simulink model "Boeing787_debug"  (R2013a)
settings: Solver=ode23tb  SolverMode=SingleTasking  StartTime=0.0  StopTime=18000  RelTol=1e-3
InitFcn:
  | load('SampleOutput.mat')
  | 
  | load('SampleFuelBurn.mat')
StartFcn:
  | tic
StopFcn:
  | ttt = toc
  | tend = eval(get_param(bdroot,'StopTime'));
  | disp(['Total Simulation Time (s) = ' num2str(ttt) 's']);
  | RTR =  ttt/tend
  | disp(['Simulation Speed is ' num2str(tend/ttt) 'x faster than real-time']);
values from neighbouring files (symbols this model uses):
  FuelBurn = [0 0 0 0 0 0 0 0 0 0 0 0 ... (18249 elements, 1x18249)]    [Benchmark_data1.mat]
undefined symbols (not defined in the file or in its folder): CurrentMission, seed
libraries: PowerFlowLib x20, simulink x14, powerlib_meascontrol x3
(part 17 of 17)

== system Boeing787_debug/Electrical/Generation Unit Sync-Sync4/Generator/Generator Power Loss ==
  Ed : Inport
  Eq : Inport  Port=2
  Id : Inport  Port=3
  Iq : Inport  Port=4
  Te : Inport  Port=5
  w/ws : Inport  Port=6
  Bus Creator : BusCreator  Inputs=6
  Gain1 : Gain  Gain=SB
  Gain2 : Gain  Gain=SB
  Gain3 : Gain  Gain=SB
  Product : Product  RndMeth=Zero
  Product1 : Product  RndMeth=Zero
  Product2 : Product  RndMeth=Zero
  Sum1 : Sum  Inputs=-+
  Sum2 : Sum
  PE : Outport
  PM : Outport  Port=2
  PLOSS : Outport  Port=3
  m : Outport  Port=4
  wires:
  Ed/1 -> [Ed]
  Eq/1 -> [Eq]
  Id/1 -> [Id]
  Iq/1 -> [Iq]
  Te/1 -> [Te]
  w/ws/1 -> [nu]
  [Ed] -> Product/1
  [Id] -> Product/2
  [Eq] -> Product1/1
  [Iq] -> Product1/2
  [Te] -> Product2/1
  [nu] -> Product2/2
  Product/1 -> Sum2/1
  Product1/1 -> Sum2/2
  Sum2/1 -> Sum1/1, Gain1/1
  Product2/1 -> Sum1/2, Gain3/1
  Sum1/1 -> Gain2/1
  [Ed] -> Bus Creator/1  "Vd"
  [Id] -> Bus Creator/2  "Id"
  [Eq] -> Bus Creator/3  "Vq"
  [Iq] -> Bus Creator/4  "Iq"
  [Te] -> Bus Creator/5  "Te"
  [nu] -> Bus Creator/6  "nu"
  Bus Creator/1 -> m/1
  Gain2/1 -> PLOSS/1
  Gain1/1 -> PE/1
  Gain3/1 -> PM/1

== system Boeing787_debug/Electrical/Generation Unit Sync-Sync4/Generator/Stator Voltage ==
  Id : Inport
  Iq : Inport  Port=2
  Eq1 : Inport  Port=3
  Ed1 : Inport  Port=4
  Phi_1d : Inport  Port=5
  Phi_2q : Inport  Port=6
  w/ws : Inport  Port=7
  Temp : Inport  Port=8
  Gain : Gain  Gain=(Xq2 - Xls)/(Xq1 - Xls)
  Gain1 : Gain  Gain=(Xq1 - Xq2)/(Xq1 - Xls)
  Gain2 : Gain  Gain=(Xq2 - Xd2)
  Gain3 : Gain  Gain=(Xd2 - Xls)/(Xd1 - Xls)
  Gain4 : Gain  Gain=(Xd1 - Xd2)/(Xd1 - Xls)
  Gain5 : Gain  Gain=Rs
  Gain6 : Gain  Gain=Xd2
  Gain7 : Gain  Gain=Rs
  Gain8 : Gain  Gain=Xd2
  Product{,1..3,5} (5 alike) : Product  RndMeth=Zero
  Product4 : Product
  Sum : Sum
  Sum1 : Sum  Inputs=+-+
  Sum2 : Sum  Inputs=--+
  Sum3 : Sum  Inputs=-++
  Ed : Outport
  Eq : Outport  Port=2
  wires:
  Iq/1 -> Gain6/1, Product5/2, Gain2/1
  Product5/1 -> Gain7/1
  Product4/1 -> Sum3/1
  Gain5/1 -> Product4/1
  Temp/1 -> Product4/2, Product5/1
  Gain2/1 -> Sum1/3
  Ed1/1 -> Gain/1
  Phi_2q/1 -> Gain1/1
  Eq1/1 -> Gain3/1
  Phi_1d/1 -> Gain4/1
  Gain4/1 -> Sum/2
  Gain3/1 -> Sum/1
  Gain/1 -> Sum1/1
  Gain1/1 -> Sum1/2
  Sum/1 -> Product/1
  Sum1/1 -> Product1/1
  w/ws/1 -> Product1/2, Product/2, Product3/2, Product2/1
  Product/1 -> Sum2/3
  Id/1 -> Gain5/1, Gain8/1
  Gain6/1 -> Product2/2
  Gain8/1 -> Product3/1
  Product1/1 -> Sum3/2
  Product2/1 -> Sum3/3
  Sum3/1 -> Ed/1  "Vd"
  Sum2/1 -> Eq/1  "Vq"
  Product3/1 -> Sum2/1
  Gain7/1 -> Sum2/2

== system Boeing787_debug/Electrical/Generation Unit Sync-Sync5/Exciter/Dynamics ==
  Id : Inport
  Iq : Inport  Port=2
  Efd : Inport  Port=3
  Temp : Inport  Port=4
  Gain : Gain  Gain=Xd1_exc - Xls_exc
  Gain1 : Gain  Gain=(Xd1_exc - Xd2_exc)/(Xd1_exc-Xls_exc)^2
  Gain10 : Gain  Gain=Xq1_exc - Xls_exc
  Gain11 : Gain  Gain=1/Tqo2_exc
  Gain2 : Gain  Gain=Xd_exc - Xd1_exc
  Gain3 : Gain  Gain=1/Tdo1_exc
  Gain4 : Gain  Gain=Xq1_exc - Xls_exc
  Gain5 : Gain  Gain=(Xq1_exc - Xq2_exc)/(Xq1_exc - Xls_exc)^2
  Gain6 : Gain  Gain=Xq_exc - Xq1_exc
  Gain7 : Gain  Gain=1/Tqo1_exc
  Gain8 : Gain  Gain=Xd1_exc - Xls_exc
  Gain9 : Gain  Gain=1/Tdo2_exc
  Integrator{,1..3} (4 alike) : Integrator
  Product{,1..3} (4 alike) : Product
  Sum : Sum  Inputs=++-
  Sum1 : Sum  Inputs=+-
  Sum2 : Sum  Inputs=--+
  Sum3 : Sum  Inputs=+++
  Sum4 : Sum  Inputs=+-
  Sum5 : Sum  Inputs=-+
  Sum6 : Sum  Inputs=--+
  Sum7 : Sum  Inputs=---
  Eq1 : Outport
  Ed1 : Outport  Port=2
  Phi_1d : Outport  Port=3
  Phi_2q : Outport  Port=4
  wires:
  Integrator/1 -> Eq1/1, [Eq1]
  [Id] -> Gain/1
  Gain/1 -> Sum/1
  [Phi_1d] -> Sum/2
  [Eq1] -> Sum/3
  Sum/1 -> Gain1/1
  [Id] -> Sum1/1
  Gain1/1 -> Sum1/2
  Sum1/1 -> Gain2/1
  [Eq1] -> Sum2/1
  Gain2/1 -> Sum2/2
  [Efd] -> Sum2/3
  Sum2/1 -> Gain3/1
  Integrator1/1 -> Ed1/1, [Ed1]
  [Iq] -> Gain4/1
  Gain4/1 -> Sum3/1
  [Phi_2q] -> Sum3/2
  [Ed1] -> Sum3/3
  Sum3/1 -> Gain5/1
  [Iq] -> Sum4/1
  Gain5/1 -> Sum4/2
  Sum4/1 -> Gain6/1
  [Ed1] -> Sum5/1
  Gain6/1 -> Sum5/2
  Sum5/1 -> Gain7/1
  [Id] -> Gain8/1
  Gain8/1 -> Sum6/1
  [Phi_1d] -> Sum6/2
  [Eq1] -> Sum6/3
  Sum6/1 -> Gain9/1
  Integrator2/1 -> [Phi_1d], Phi_1d/1
  [Iq] -> Gain10/1
  Gain10/1 -> Sum7/1
  [Phi_2q] -> Sum7/2
  [Ed1] -> Sum7/3
  Sum7/1 -> Gain11/1
  Integrator3/1 -> [Phi_2q], Phi_2q/1
  Id/1 -> [Id]
  Iq/1 -> [Iq]
  Efd/1 -> [Efd]
  Temp/1 -> [R_temp_delta]
  Gain3/1 -> Product/2
  Product/1 -> Integrator/1
  [R_temp_delta] -> Product/1
  [R_temp_delta] -> Product1/1
  Gain7/1 -> Product1/2
  Product1/1 -> Integrator1/1
  [R_temp_delta] -> Product2/1
  Gain11/1 -> Product2/2
  Product2/1 -> Integrator3/1
  [R_temp_delta] -> Product3/1
  Gain9/1 -> Product3/2
  Product3/1 -> Integrator2/1

== system Boeing787_debug/Electrical/Generation Unit Sync-Sync5/Exciter/Electromagnetic Torque Output Power ==
  note: Torque from Field Winding
  note: Torque from Damper Windings
  Id : Inport
  Iq : Inport  Port=2
  Eq1 : Inport  Port=3
  Ed1 : Inport  Port=4
  Phi_1d : Inport  Port=5
  Phi_2q : Inport  Port=6
  Gain : Gain  Gain=(Xd2_exc - Xls_exc)/(Xd1_exc - Xls_exc)
  Gain1 : Gain  Gain=(Xq2_exc - Xls_exc)/(Xq1_exc - Xls_exc)
  Gain2 : Gain  Gain=(Xd1_exc - Xd2_exc)/(Xd1_exc-Xls_exc)
  Gain3 : Gain  Gain=(Xq1_exc - Xq2_exc)/(Xq1_exc-Xls_exc)
  Gain4 : Gain  Gain=(Xq2_exc - Xd2_exc)
  Product{,1..4} (5 alike) : Product  RndMeth=Zero
  Sum : Sum
  Sum1 : Sum  Inputs=+-+
  Sum2 : Sum
  TE : Outport
  wires:
  Id/1 -> [Id]
  Eq1/1 -> [Eq1]
  Ed1/1 -> [Ed1]
  Phi_1d/1 -> [Phi_1d]
  Phi_2q/1 -> [Phi_2q]
  Iq/1 -> [Iq]
  [Eq1] -> Product/1
  [Iq] -> Product/2
  Product/1 -> Gain/1
  [Ed1] -> Product1/1
  [Id] -> Product1/2
  Product1/1 -> Gain1/1
  [Iq] -> Product2/1
  [Phi_1d] -> Product2/2
  Product2/1 -> Gain2/1
  [Id] -> Product3/1
  [Phi_2q] -> Product3/2
  Product3/1 -> Gain3/1
  [Id] -> Product4/1
  [Iq] -> Product4/2
  Product4/1 -> Gain4/1
  Gain3/1 -> Sum1/2
  Gain2/1 -> Sum1/1
  Gain4/1 -> Sum1/3
  Gain/1 -> Sum/1
  Gain1/1 -> Sum/2
  Sum/1 -> Sum2/1
  Sum1/1 -> Sum2/2
  Sum2/1 -> TE/1

== system Boeing787_debug/Electrical/Generation Unit Sync-Sync5/Exciter/Generator Power Loss ==
  Ed : Inport
  Eq : Inport  Port=2
  Id : Inport  Port=3
  Iq : Inport  Port=4
  Te : Inport  Port=5
  w/ws : Inport  Port=6
  Bus Creator : BusCreator  Inputs=6
  Gain1 : Gain  Gain=SB_exc
  Gain2 : Gain  Gain=SB_exc
  Gain3 : Gain  Gain=SB_exc
  Product : Product  RndMeth=Zero
  Product1 : Product  RndMeth=Zero
  Product2 : Product  RndMeth=Zero
  Sum1 : Sum  Inputs=-+
  Sum2 : Sum
  PE : Outport
  PM : Outport  Port=2
  PLOSS : Outport  Port=3
  m : Outport  Port=4
  wires:
  Ed/1 -> [Ed]
  Eq/1 -> [Eq]
  Id/1 -> [Id]
  Iq/1 -> [Iq]
  Te/1 -> [Te]
  w/ws/1 -> [nu]
  [Ed] -> Product/1
  [Id] -> Product/2
  [Eq] -> Product1/1
  [Iq] -> Product1/2
  [Te] -> Product2/1
  [nu] -> Product2/2
  Product/1 -> Sum2/1
  Product1/1 -> Sum2/2
  Sum2/1 -> Sum1/1, Gain1/1
  Product2/1 -> Sum1/2, Gain3/1
  Sum1/1 -> Gain2/1
  [Ed] -> Bus Creator/1  "Vd"
  [Id] -> Bus Creator/2  "Id"
  [Eq] -> Bus Creator/3  "Vq"
  [Iq] -> Bus Creator/4  "Iq"
  [Te] -> Bus Creator/5  "Te"
  [nu] -> Bus Creator/6  "nu"
  Bus Creator/1 -> m/1
  Gain2/1 -> PLOSS/1
  Gain1/1 -> PE/1
  Gain3/1 -> PM/1

== system Boeing787_debug/Electrical/Generation Unit Sync-Sync5/Exciter/Stator Voltage ==
  Id : Inport
  Iq : Inport  Port=2
  Eq1 : Inport  Port=3
  Ed1 : Inport  Port=4
  Phi_1d : Inport  Port=5
  Phi_2q : Inport  Port=6
  w/ws : Inport  Port=7
  Temp : Inport  Port=8
  Gain : Gain  Gain=(Xq2_exc - Xls_exc)/(Xq1_exc - Xls_exc)
  Gain1 : Gain  Gain=(Xq1_exc - Xq2_exc)/(Xq1_exc - Xls_exc)
  Gain2 : Gain  Gain=(Xq2_exc - Xd2_exc)
  Gain3 : Gain  Gain=(Xd2_exc - Xls_exc)/(Xd1_exc - Xls_exc)
  Gain4 : Gain  Gain=(Xd1_exc - Xd2_exc)/(Xd1_exc - Xls_exc)
  Gain5 : Gain  Gain=Rs_exc
  Gain6 : Gain  Gain=Xd2+XTL
  Gain7 : Gain  Gain=Rs_exc+RTL_exc
  Gain8 : Gain  Gain=Xd2_exc+XTL_exc
  Product{,1..3,5} (5 alike) : Product  RndMeth=Zero
  Product4 : Product
  Sum : Sum
  Sum1 : Sum  Inputs=+-+
  Sum2 : Sum  Inputs=--+
  Sum3 : Sum  Inputs=-++
  Ed : Outport
  Eq : Outport  Port=2
  wires:
  Ed1/1 -> Gain/1
  Phi_2q/1 -> Gain1/1
  Iq/1 -> Product5/2, Gain6/1, Gain2/1
  Eq1/1 -> Gain3/1
  Phi_1d/1 -> Gain4/1
  Gain4/1 -> Sum/2
  Gain3/1 -> Sum/1
  Gain/1 -> Sum1/1
  Gain1/1 -> Sum1/2
  Sum/1 -> Product/1
  Sum1/1 -> Product1/1
  w/ws/1 -> Product1/2, Product/2, Product3/2, Product2/1
  Product/1 -> Sum2/3
  Id/1 -> Gain5/1, Gain8/1
  Gain6/1 -> Product2/2
  Gain8/1 -> Product3/1
  Product1/1 -> Sum3/2
  Gain2/1 -> Sum1/3
  Product2/1 -> Sum3/3
  Sum3/1 -> Ed/1  "Vd"
  Sum2/1 -> Eq/1  "Vq"
  Product3/1 -> Sum2/1
  Gain7/1 -> Sum2/2
  Product4/1 -> Sum3/1
  Gain5/1 -> Product4/1
  Temp/1 -> Product5/1, Product4/2
  Product5/1 -> Gain7/1

== system Boeing787_debug/Electrical/Generation Unit Sync-Sync5/Generator/Dynamics ==
  Id : Inport
  Iq : Inport  Port=2
  Efd : Inport  Port=3
  Temp : Inport  Port=4
  Gain : Gain  Gain=Xd1 - Xls
  Gain1 : Gain  Gain=(Xd1 - Xd2)/(Xd1-Xls)^2
  Gain10 : Gain  Gain=Xq1 - Xls
  Gain11 : Gain  Gain=1/Tqo2
  Gain2 : Gain  Gain=Xd - Xd1
  Gain3 : Gain  Gain=1/Tdo1
  Gain4 : Gain  Gain=Xq1 - Xls
  Gain5 : Gain  Gain=(Xq1 - Xq2)/(Xq1 - Xls)^2
  Gain6 : Gain  Gain=Xq - Xq1
  Gain7 : Gain  Gain=1/Tqo1
  Gain8 : Gain  Gain=Xd1 - Xls
  Gain9 : Gain  Gain=1/Tdo2
  Integrator{,1..3} (4 alike) : Integrator
  Product{1..4} (4 alike) : Product
  Sum : Sum  Inputs=++-
  Sum1 : Sum  Inputs=+-
  Sum2 : Sum  Inputs=--+
  Sum3 : Sum  Inputs=+++
  Sum4 : Sum  Inputs=+-
  Sum5 : Sum  Inputs=-+
  Sum6 : Sum  Inputs=--+
  Sum7 : Sum  Inputs=---
  Eq1 : Outport
  Ed1 : Outport  Port=2
  Phi_1d : Outport  Port=3
  Phi_2q : Outport  Port=4
  wires:
  Efd/1 -> [Efd]
  Iq/1 -> [Iq]
  Id/1 -> [Id]
  Integrator3/1 -> Phi_2q/1, [Phi_2q]
  Sum7/1 -> Gain11/1
  [Ed1] -> Sum7/3
  [Phi_2q] -> Sum7/2
  Gain10/1 -> Sum7/1
  [Iq] -> Gain10/1
  Integrator2/1 -> Phi_1d/1, [Phi_1d]
  Sum6/1 -> Gain9/1
  [Eq1] -> Sum6/3
  [Phi_1d] -> Sum6/2
  Gain8/1 -> Sum6/1
  [Id] -> Gain8/1
  Sum5/1 -> Gain7/1
  Gain6/1 -> Sum5/2
  [Ed1] -> Sum5/1
  Sum4/1 -> Gain6/1
  Gain5/1 -> Sum4/2
  [Iq] -> Sum4/1
  Sum3/1 -> Gain5/1
  [Ed1] -> Sum3/3
  [Phi_2q] -> Sum3/2
  Gain4/1 -> Sum3/1
  [Iq] -> Gain4/1
  Integrator1/1 -> [Ed1], Ed1/1
  Sum2/1 -> Gain3/1
  [Efd] -> Sum2/3
  Gain2/1 -> Sum2/2
  [Eq1] -> Sum2/1
  Sum1/1 -> Gain2/1
  Gain1/1 -> Sum1/2
  [Id] -> Sum1/1
  Sum/1 -> Gain1/1
  [Eq1] -> Sum/3
  [Id] -> Gain/1
  Integrator/1 -> [Eq1], Eq1/1
  Gain/1 -> Sum/1
  [Phi_1d] -> Sum/2
  Temp/1 -> [R_temp_delta]
  [R_temp_delta] -> Product3/1
  Gain9/1 -> Product3/2
  Product3/1 -> Integrator2/1
  [R_temp_delta] -> Product1/1
  Gain11/1 -> Product1/2
  Product1/1 -> Integrator3/1
  [R_temp_delta] -> Product2/1
  Gain3/1 -> Product2/2
  Product2/1 -> Integrator/1
  [R_temp_delta] -> Product4/1
  Gain7/1 -> Product4/2
  Product4/1 -> Integrator1/1

== system Boeing787_debug/Electrical/Generation Unit Sync-Sync5/Generator/Electromagnetic Torque Output Power ==
  note: Torque from Damper Windings
  note: Torque from Field Winding
  Id : Inport
  Iq : Inport  Port=2
  Eq1 : Inport  Port=3
  Ed1 : Inport  Port=4
  Phi_1d : Inport  Port=5
  Phi_2q : Inport  Port=6
  Gain : Gain  Gain=(Xd2 - Xls)/(Xd1 - Xls)
  Gain1 : Gain  Gain=(Xq2 - Xls)/(Xq1 - Xls)
  Gain2 : Gain  Gain=(Xd1 - Xd2)/(Xd1-Xls)
  Gain3 : Gain  Gain=(Xq1 - Xq2)/(Xq1-Xls)
  Gain4 : Gain  Gain=(Xq2 - Xd2)
  Product{,1..4} (5 alike) : Product  RndMeth=Zero
  Scope{,1..4} (5 alike) : Scope
      Scope settings: YMin=-0.00574  YMax=0.05167  SaveName=ScopeData2
      Scope1 settings: YMin=-0.04047  YMax=0.36422  SaveName=ScopeData3
      Scope2 settings: YMin=-0.001  YMax=0.00903  SaveName=ScopeData4
      Scope3 settings: YMin=-0.00634  YMax=0.0007  SaveName=ScopeData5
      Scope4 settings: YMin=0.06667  YMax=0.26667  SaveName=ScopeData6
  Sum : Sum
  Sum1 : Sum  Inputs=+-+
  Sum2 : Sum
  TE : Outport
  wires:
  [Eq1] -> Product/1, Scope1/1
  Sum2/1 -> TE/1
  Sum1/1 -> Sum2/2
  Sum/1 -> Sum2/1
  Gain1/1 -> Sum/2
  Gain/1 -> Sum/1, Scope/1
  Gain4/1 -> Sum1/3
  Gain2/1 -> Scope2/1, Sum1/1
  Gain3/1 -> Sum1/2
  Product4/1 -> Gain4/1
  [Iq] -> Product4/2
  [Id] -> Product4/1
  Product3/1 -> Gain3/1
  [Phi_2q] -> Product3/2
  [Id] -> Product3/1
  Product2/1 -> Gain2/1
  [Phi_1d] -> Product2/2
  [Iq] -> Product2/1
  Product1/1 -> Gain1/1
  [Id] -> Product1/2
  [Ed1] -> Product1/1
  Product/1 -> Gain/1, Scope3/1
  [Iq] -> Product/2, Scope4/1
  Iq/1 -> [Iq]
  Phi_2q/1 -> [Phi_2q]
  Phi_1d/1 -> [Phi_1d]
  Ed1/1 -> [Ed1]
  Eq1/1 -> [Eq1]
  Id/1 -> [Id]

== system Boeing787_debug/Electrical/Generation Unit Sync-Sync5/Generator/Generator Power Loss ==
  Ed : Inport
  Eq : Inport  Port=2
  Id : Inport  Port=3
  Iq : Inport  Port=4
  Te : Inport  Port=5
  w/ws : Inport  Port=6
  Bus Creator : BusCreator  Inputs=6
  Gain1 : Gain  Gain=SB
  Gain2 : Gain  Gain=SB
  Gain3 : Gain  Gain=SB
  Product : Product  RndMeth=Zero
  Product1 : Product  RndMeth=Zero
  Product2 : Product  RndMeth=Zero
  Sum1 : Sum  Inputs=-+
  Sum2 : Sum
  PE : Outport
  PM : Outport  Port=2
  PLOSS : Outport  Port=3
  m : Outport  Port=4
  wires:
  Gain3/1 -> PM/1
  Gain1/1 -> PE/1
  Gain2/1 -> PLOSS/1
  Bus Creator/1 -> m/1
  [nu] -> Bus Creator/6  "nu"
  [Te] -> Bus Creator/5  "Te"
  [Iq] -> Bus Creator/4  "Iq"
  [Eq] -> Bus Creator/3  "Vq"
  [Id] -> Bus Creator/2  "Id"
  [Ed] -> Bus Creator/1  "Vd"
  Sum1/1 -> Gain2/1
  Product2/1 -> Gain3/1, Sum1/2
  Sum2/1 -> Gain1/1, Sum1/1
  Product1/1 -> Sum2/2
  Product/1 -> Sum2/1
  [nu] -> Product2/2
  [Te] -> Product2/1
  [Iq] -> Product1/2
  [Eq] -> Product1/1
  [Id] -> Product/2
  [Ed] -> Product/1
  w/ws/1 -> [nu]
  Te/1 -> [Te]
  Iq/1 -> [Iq]
  Id/1 -> [Id]
  Eq/1 -> [Eq]
  Ed/1 -> [Ed]

== system Boeing787_debug/Electrical/Generation Unit Sync-Sync5/Generator/Stator Voltage ==
  Id : Inport
  Iq : Inport  Port=2
  Eq1 : Inport  Port=3
  Ed1 : Inport  Port=4
  Phi_1d : Inport  Port=5
  Phi_2q : Inport  Port=6
  w/ws : Inport  Port=7
  Temp : Inport  Port=8
  Gain : Gain  Gain=(Xq2 - Xls)/(Xq1 - Xls)
  Gain1 : Gain  Gain=(Xq1 - Xq2)/(Xq1 - Xls)
  Gain2 : Gain  Gain=(Xq2 - Xd2)
  Gain3 : Gain  Gain=(Xd2 - Xls)/(Xd1 - Xls)
  Gain4 : Gain  Gain=(Xd1 - Xd2)/(Xd1 - Xls)
  Gain5 : Gain  Gain=Rs
  Gain6 : Gain  Gain=Xd2
  Gain7 : Gain  Gain=Rs
  Gain8 : Gain  Gain=Xd2
  Product{,1..3,5} (5 alike) : Product  RndMeth=Zero
  Product4 : Product
  Sum : Sum
  Sum1 : Sum  Inputs=+-+
  Sum2 : Sum  Inputs=--+
  Sum3 : Sum  Inputs=-++
  Ed : Outport
  Eq : Outport  Port=2
  wires:
  Gain7/1 -> Sum2/2
  Product3/1 -> Sum2/1
  Sum2/1 -> Eq/1  "Vq"
  Sum3/1 -> Ed/1  "Vd"
  Product2/1 -> Sum3/3
  Product1/1 -> Sum3/2
  Gain8/1 -> Product3/1
  Gain6/1 -> Product2/2
  Id/1 -> Gain8/1, Gain5/1
  Product/1 -> Sum2/3
  w/ws/1 -> Product2/1, Product3/2, Product/2, Product1/2
  Sum1/1 -> Product1/1
  Sum/1 -> Product/1
  Gain1/1 -> Sum1/2
  Gain/1 -> Sum1/1
  Gain3/1 -> Sum/1
  Gain4/1 -> Sum/2
  Phi_1d/1 -> Gain4/1
  Eq1/1 -> Gain3/1
  Phi_2q/1 -> Gain1/1
  Ed1/1 -> Gain/1
  Gain2/1 -> Sum1/3
  Temp/1 -> Product5/1, Product4/2
  Gain5/1 -> Product4/1
  Product4/1 -> Sum3/1
  Product5/1 -> Gain7/1
  Iq/1 -> Gain2/1, Product5/2, Gain6/1

== matlab function Boeing787_debug/Electrical/Thermal Interface/Generator 2 Thermal Model/MATLAB Function ==
  data: Ploss input; Tdot output; Tf input; Ta input; mdot_f input; Tgen input
function Tdot = Generator_loss(Ploss, Tf, Ta, mdot_f, Tgen)
%% Constants

% generator parameters
Cp_gen  = 0.49*1000;                     % Cp of carbon steel [J/kg-K]
m_gen   = 250;                        % mass of generator [kg]
L_gen   = 0.5;                        % length of generator [m]
D_gen   = 0.3;                        % diameter of generator [m]

% fuel parameters
nu_f    = 4.77*10^-6;                    % kinematic viscosity of JP8 [m^2/s]
k_f     = 0.115;                         % thermal conductivity of JP8[W/m-K]
rho_f   = 900;                           % density [kg/m^3]
Cp_f    = 1900;                          % Cp of Jp8 [J/kg-K]

% air parameters
nu_a    = 1.568*10^-5;                   % kinematic viscosity of air [m^2/s]
k_a     = 0.0257;                        % thermal conductivity of air[W/m-K]
rho_a   = 1.205;                         % density [kg/m^3]
Cp_a    = 1005;                          % Cp of Jp8 [J/kg-K]


% outer surface area of generator
A_a   = pi*D_gen*L_gen + 2*pi/4*D_gen^2;

% assume the inner surface area for the water jacket is a series of tubes
nTubes = 15;                        % number of tubes
D_tubes = .02;                      % diameter of tubes [m]

A_f   = nTubes*(pi*D_tubes*L_gen);  % surface area of fuel interactions

%% Calculations
% fuel
V_f = mdot_f / rho_f / (D_tubes^2/4*pi); 

Pr_f = rho_f * nu_f * Cp_f / k_f;
Re_f = V_f * L_gen / nu_f;

h_f = 0.037 * Re_f^(4/5) * Pr_f^(1/3) * k_f / L_gen;

% air
V_a = 3; % assume free stream velocity is 3m/s

Pr_a = rho_a * nu_a * Cp_a / k_a;
Re_a = V_a * L_gen / nu_a;

h_a = 0.037 * Re_a^(4/5) * Pr_a^(1/3) * k_a / L_gen;




Tdot = 1/(m_gen*Cp_gen) * ( Ploss + (Tf - Tgen)*h_f*A_f + (Ta - Tgen)*h_a*A_a);

== matlab function Boeing787_debug/Electrical/Thermal Interface/Generator 1 Thermal Model/MATLAB Function ==
  data: Ploss input; Tdot output; Tf input; Ta input; mdot_f input; Tgen input
function Tdot = Generator_loss(Ploss, Tf, Ta, mdot_f, Tgen)
%% Constants

% generator parameters
Cp_gen  = 0.49*1000;                     % Cp of carbon steel [J/kg-K]
m_gen   = 250;                        % mass of generator [kg]
L_gen   = 0.5;                        % length of generator [m]
D_gen   = 0.3;                        % diameter of generator [m]

% fuel parameters
nu_f    = 4.77*10^-6;                    % kinematic viscosity of JP8 [m^2/s]
k_f     = 0.115;                         % thermal conductivity of JP8[W/m-K]
rho_f   = 900;                           % density [kg/m^3]
Cp_f    = 1900;                          % Cp of Jp8 [J/kg-K]

% air parameters
nu_a    = 1.568*10^-5;                   % kinematic viscosity of air [m^2/s]
k_a     = 0.0257;                        % thermal conductivity of air[W/m-K]
rho_a   = 1.205;                         % density [kg/m^3]
Cp_a    = 1005;                          % Cp of Jp8 [J/kg-K]


% outer surface area of generator
A_a   = pi*D_gen*L_gen + 2*pi/4*D_gen^2;

% assume the inner surface area for the water jacket is a series of tubes
nTubes = 15;                        % number of tubes
D_tubes = .02;                      % diameter of tubes [m]

A_f   = nTubes*(pi*D_tubes*L_gen);  % surface area of fuel interactions

%% Calculations
% fuel
V_f = mdot_f / rho_f / (D_tubes^2/4*pi); 

Pr_f = rho_f * nu_f * Cp_f / k_f;
Re_f = V_f * L_gen / nu_f;

h_f = 0.037 * Re_f^(4/5) * Pr_f^(1/3) * k_f / L_gen;

% air
V_a = 3; % assume free stream velocity is 3m/s

Pr_a = rho_a * nu_a * Cp_a / k_a;
Re_a = V_a * L_gen / nu_a;

h_a = 0.037 * Re_a^(4/5) * Pr_a^(1/3) * k_a / L_gen;




Tdot = 1/(m_gen*Cp_gen) * ( Ploss + (Tf - Tgen)*h_f*A_f + (Ta - Tgen)*h_a*A_a);

== matlab function Boeing787_debug/Electrical/Thermal Interface/Generator 3 Thermal Model/MATLAB Function ==
  data: Ploss input; Tdot output; Tf input; Ta input; mdot_f input; Tgen input
function Tdot = Generator_loss(Ploss, Tf, Ta, mdot_f, Tgen)
%% Constants

% generator parameters
Cp_gen  = 0.49*1000;                     % Cp of carbon steel [J/kg-K]
m_gen   = 250;                        % mass of generator [kg]
L_gen   = 0.5;                        % length of generator [m]
D_gen   = 0.3;                        % diameter of generator [m]

% fuel parameters
nu_f    = 4.77*10^-6;                    % kinematic viscosity of JP8 [m^2/s]
k_f     = 0.115;                         % thermal conductivity of JP8[W/m-K]
rho_f   = 900;                           % density [kg/m^3]
Cp_f    = 1900;                          % Cp of Jp8 [J/kg-K]

% air parameters
nu_a    = 1.568*10^-5;                   % kinematic viscosity of air [m^2/s]
k_a     = 0.0257;                        % thermal conductivity of air[W/m-K]
rho_a   = 1.205;                         % density [kg/m^3]
Cp_a    = 1005;                          % Cp of Jp8 [J/kg-K]


% outer surface area of generator
A_a   = pi*D_gen*L_gen + 2*pi/4*D_gen^2;

% assume the inner surface area for the water jacket is a series of tubes
nTubes = 15;                        % number of tubes
D_tubes = .02;                      % diameter of tubes [m]

A_f   = nTubes*(pi*D_tubes*L_gen);  % surface area of fuel interactions

%% Calculations
% fuel
V_f = mdot_f / rho_f / (D_tubes^2/4*pi); 

Pr_f = rho_f * nu_f * Cp_f / k_f;
Re_f = V_f * L_gen / nu_f;

h_f = 0.037 * Re_f^(4/5) * Pr_f^(1/3) * k_f / L_gen;

% air
V_a = 3; % assume free stream velocity is 3m/s

Pr_a = rho_a * nu_a * Cp_a / k_a;
Re_a = V_a * L_gen / nu_a;

h_a = 0.037 * Re_a^(4/5) * Pr_a^(1/3) * k_a / L_gen;




Tdot = 1/(m_gen*Cp_gen) * ( Ploss + (Tf - Tgen)*h_f*A_f + (Ta - Tgen)*h_a*A_a);

== matlab function Boeing787_debug/Electrical/Thermal Interface/Generator 4 Thermal Model/MATLAB Function ==
  data: Ploss input; Tdot output; Tf input; Ta input; mdot_f input; Tgen input
function Tdot = Generator_loss(Ploss, Tf, Ta, mdot_f, Tgen)
%% Constants

% generator parameters
Cp_gen  = 0.49*1000;                     % Cp of carbon steel [J/kg-K]
m_gen   = 250;                        % mass of generator [kg]
L_gen   = 0.5;                        % length of generator [m]
D_gen   = 0.3;                        % diameter of generator [m]

% fuel parameters
nu_f    = 4.77*10^-6;                    % kinematic viscosity of JP8 [m^2/s]
k_f     = 0.115;                         % thermal conductivity of JP8[W/m-K]
rho_f   = 900;                           % density [kg/m^3]
Cp_f    = 1900;                          % Cp of Jp8 [J/kg-K]

% air parameters
nu_a    = 1.568*10^-5;                   % kinematic viscosity of air [m^2/s]
k_a     = 0.0257;                        % thermal conductivity of air[W/m-K]
rho_a   = 1.205;                         % density [kg/m^3]
Cp_a    = 1005;                          % Cp of Jp8 [J/kg-K]


% outer surface area of generator
A_a   = pi*D_gen*L_gen + 2*pi/4*D_gen^2;

% assume the inner surface area for the water jacket is a series of tubes
nTubes = 15;                        % number of tubes
D_tubes = .02;                      % diameter of tubes [m]

A_f   = nTubes*(pi*D_tubes*L_gen);  % surface area of fuel interactions

%% Calculations
% fuel
V_f = mdot_f / rho_f / (D_tubes^2/4*pi); 

Pr_f = rho_f * nu_f * Cp_f / k_f;
Re_f = V_f * L_gen / nu_f;

h_f = 0.037 * Re_f^(4/5) * Pr_f^(1/3) * k_f / L_gen;

% air
V_a = 3; % assume free stream velocity is 3m/s

Pr_a = rho_a * nu_a * Cp_a / k_a;
Re_a = V_a * L_gen / nu_a;

h_a = 0.037 * Re_a^(4/5) * Pr_a^(1/3) * k_a / L_gen;




Tdot = 1/(m_gen*Cp_gen) * ( Ploss + (Tf - Tgen)*h_f*A_f + (Ta - Tgen)*h_a*A_a);

== matlab function Boeing787_debug/Electrical/Thermal Interface/Generator 5 Thermal Model/MATLAB Function ==
  data: Ploss input; Tdot output; Tf input; Ta input; mdot_f input; Tgen input
function Tdot = Generator_loss(Ploss, Tf, Ta, mdot_f, Tgen)
%% Constants

% generator parameters
Cp_gen  = 0.49*1000;                     % Cp of carbon steel [J/kg-K]
m_gen   = 250;                        % mass of generator [kg]
L_gen   = 0.5;                        % length of generator [m]
D_gen   = 0.3;                        % diameter of generator [m]

% fuel parameters
nu_f    = 4.77*10^-6;                    % kinematic viscosity of JP8 [m^2/s]
k_f     = 0.115;                         % thermal conductivity of JP8[W/m-K]
rho_f   = 900;                           % density [kg/m^3]
Cp_f    = 1900;                          % Cp of Jp8 [J/kg-K]

% air parameters
nu_a    = 1.568*10^-5;                   % kinematic viscosity of air [m^2/s]
k_a     = 0.0257;                        % thermal conductivity of air[W/m-K]
rho_a   = 1.205;                         % density [kg/m^3]
Cp_a    = 1005;                          % Cp of Jp8 [J/kg-K]


% outer surface area of generator
A_a   = pi*D_gen*L_gen + 2*pi/4*D_gen^2;

% assume the inner surface area for the water jacket is a series of tubes
nTubes = 15;                        % number of tubes
D_tubes = .02;                      % diameter of tubes [m]

A_f   = nTubes*(pi*D_tubes*L_gen);  % surface area of fuel interactions

%% Calculations
% fuel
V_f = mdot_f / rho_f / (D_tubes^2/4*pi); 

Pr_f = rho_f * nu_f * Cp_f / k_f;
Re_f = V_f * L_gen / nu_f;

h_f = 0.037 * Re_f^(4/5) * Pr_f^(1/3) * k_f / L_gen;

% air
V_a = 3; % assume free stream velocity is 3m/s

Pr_a = rho_a * nu_a * Cp_a / k_a;
Re_a = V_a * L_gen / nu_a;

h_a = 0.037 * Re_a^(4/5) * Pr_a^(1/3) * k_a / L_gen;




Tdot = 1/(m_gen*Cp_gen) * ( Ploss + (Tf - Tgen)*h_f*A_f + (Ta - Tgen)*h_a*A_a);

== matlab function Boeing787_debug/Electrical/Thermal Interface/Generator 6 Thermal Model/MATLAB Function ==
  data: Ploss input; Tdot output; Tf input; Ta input; mdot_f input; Tgen input
function Tdot = Generator_loss(Ploss, Tf, Ta, mdot_f, Tgen)
%% Constants

% generator parameters
Cp_gen  = 0.49*1000;                     % Cp of carbon steel [J/kg-K]
m_gen   = 250;                        % mass of generator [kg]
L_gen   = 0.5;                        % length of generator [m]
D_gen   = 0.3;                        % diameter of generator [m]

% fuel parameters
nu_f    = 4.77*10^-6;                    % kinematic viscosity of JP8 [m^2/s]
k_f     = 0.115;                         % thermal conductivity of JP8[W/m-K]
rho_f   = 900;                           % density [kg/m^3]
Cp_f    = 1900;                          % Cp of Jp8 [J/kg-K]

% air parameters
nu_a    = 1.568*10^-5;                   % kinematic viscosity of air [m^2/s]
k_a     = 0.0257;                        % thermal conductivity of air[W/m-K]
rho_a   = 1.205;                         % density [kg/m^3]
Cp_a    = 1005;                          % Cp of Jp8 [J/kg-K]


% outer surface area of generator
A_a   = pi*D_gen*L_gen + 2*pi/4*D_gen^2;

% assume the inner surface area for the water jacket is a series of tubes
nTubes = 15;                        % number of tubes
D_tubes = .02;                      % diameter of tubes [m]

A_f   = nTubes*(pi*D_tubes*L_gen);  % surface area of fuel interactions

%% Calculations
% fuel
V_f = mdot_f / rho_f / (D_tubes^2/4*pi); 

Pr_f = rho_f * nu_f * Cp_f / k_f;
Re_f = V_f * L_gen / nu_f;

h_f = 0.037 * Re_f^(4/5) * Pr_f^(1/3) * k_f / L_gen;

% air
V_a = 3; % assume free stream velocity is 3m/s

Pr_a = rho_a * nu_a * Cp_a / k_a;
Re_a = V_a * L_gen / nu_a;

h_a = 0.037 * Re_a^(4/5) * Pr_a^(1/3) * k_a / L_gen;




Tdot = 1/(m_gen*Cp_gen) * ( Ploss + (Tf - Tgen)*h_f*A_f + (Ta - Tgen)*h_a*A_a);

== matlab function Boeing787_debug/Electrical/Thermal Interface/Battery Thermal Model/MATLAB Function ==
  data: Ploss input; Tdot output; Tf input; Ta input; mdot_f input; Tgen input
function Tdot = Battery_loss(Ploss, Tf, Ta, mdot_f, Tgen)
%% Constants

% generator parameters
Cp_gen  = 0.49*1000;                     % Cp of carbon steel [J/kg-K]
m_gen   = 250;                        % mass of generator [kg]
L_gen   = 0.5;                        % length of generator [m]
D_gen   = 0.3;                        % diameter of generator [m]

% fuel parameters
nu_f    = 4.77*10^-6;                    % kinematic viscosity of JP8 [m^2/s]
k_f     = 0.115;                         % thermal conductivity of JP8[W/m-K]
rho_f   = 900;                           % density [kg/m^3]
Cp_f    = 1900;                          % Cp of Jp8 [J/kg-K]

% air parameters
nu_a    = 1.568*10^-5;                   % kinematic viscosity of air [m^2/s]
k_a     = 0.0257;                        % thermal conductivity of air[W/m-K]
rho_a   = 1.205;                         % density [kg/m^3]
Cp_a    = 1005;                          % Cp of Jp8 [J/kg-K]


% outer surface area of generator
A_a   = pi*D_gen*L_gen + 2*pi/4*D_gen^2;

% assume the inner surface area for the water jacket is a series of tubes
nTubes = 15;                        % number of tubes
D_tubes = .02;                      % diameter of tubes [m]

A_f   = nTubes*(pi*D_tubes*L_gen);  % surface area of fuel interactions

%% Calculations
% fuel
V_f = mdot_f / rho_f / (D_tubes^2/4*pi); 

Pr_f = rho_f * nu_f * Cp_f / k_f;
Re_f = V_f * L_gen / nu_f;

h_f = 0.037 * Re_f^(4/5) * Pr_f^(1/3) * k_f / L_gen;

% air
V_a = 3; % assume free stream velocity is 3m/s

Pr_a = rho_a * nu_a * Cp_a / k_a;
Re_a = V_a * L_gen / nu_a;

h_a = 0.037 * Re_a^(4/5) * Pr_a^(1/3) * k_a / L_gen;




Tdot = 1/(m_gen*Cp_gen) * ( Ploss + (Tf - Tgen)*h_f*A_f + (Ta - Tgen)*h_a*A_a);

== matlab function Boeing787_debug/Electrical/Thermal Interface/Load Thermal Model/MATLAB Function ==
  data: Ploss input; Tdot output; Tf input; Ta input; mdot_f input; Tgen input
function Tdot = Generator_loss(Ploss, Tf, Ta, mdot_f, Tgen)
%% Constants

% generator parameters
Cp_gen  = 0.49*1000;                     % Cp of carbon steel [J/kg-K]
m_gen   = 250;                        % mass of generator [kg]
L_gen   = 0.5;                        % length of generator [m]
D_gen   = 0.3;                        % diameter of generator [m]

% fuel parameters
nu_f    = 4.77*10^-6;                    % kinematic viscosity of JP8 [m^2/s]
k_f     = 0.115;                         % thermal conductivity of JP8[W/m-K]
rho_f   = 900;                           % density [kg/m^3]
Cp_f    = 1900;                          % Cp of Jp8 [J/kg-K]

% air parameters
nu_a    = 1.568*10^-5;                   % kinematic viscosity of air [m^2/s]
k_a     = 0.0257;                        % thermal conductivity of air[W/m-K]
rho_a   = 1.205;                         % density [kg/m^3]
Cp_a    = 1005;                          % Cp of Jp8 [J/kg-K]


% outer surface area of generator
A_a   = pi*D_gen*L_gen + 2*pi/4*D_gen^2;

% assume the inner surface area for the water jacket is a series of tubes
nTubes = 15;                        % number of tubes
D_tubes = .02;                      % diameter of tubes [m]

A_f   = nTubes*(pi*D_tubes*L_gen);  % surface area of fuel interactions

%% Calculations
% fuel
V_f = mdot_f / rho_f / (D_tubes^2/4*pi); 

Pr_f = rho_f * nu_f * Cp_f / k_f;
Re_f = V_f * L_gen / nu_f;

h_f = 0.037 * Re_f^(4/5) * Pr_f^(1/3) * k_f / L_gen;

% air
V_a = 3; % assume free stream velocity is 3m/s

Pr_a = rho_a * nu_a * Cp_a / k_a;
Re_a = V_a * L_gen / nu_a;

h_a = 0.037 * Re_a^(4/5) * Pr_a^(1/3) * k_a / L_gen;




Tdot = 1/(m_gen*Cp_gen) * ( Ploss + (Tf - Tgen)*h_f*A_f + (Ta - Tgen)*h_a*A_a);
